simulink model "BetaMacs"  (R2023a)
settings: Solver=ode4  StartTime=0.0  StopTime=tsim  FixedStep=baseRate  RelTol=1e-6  AbsTol=1e-6
undefined symbols (not defined in the file): a1, a2, a3, b0, b1, b2, b3, baseRate, DiscIntNeverNeededParam, drop_states_ARM, drop_states_BLACK, drop_states_BLUE, drop_states_RED, F_Black_X_nominal, F_Black_Y_nominal, F_Blue_X_nominal, F_Blue_Y_nominal, F_red_X_nominal, F_red_Y_nominal, F_thrusters_BLACK, F_thrusters_BLUE, F_thrusters_RED, Gamma1_el, Gamma1_sh, Gamma1_wr, Gamma2_el, Gamma2_sh, Gamma2_wr, Gamma3_el, Gamma3_sh, Gamma3_wr, Gamma4_el, Gamma4_sh, Gamma4_wr, Gamma5_el, Gamma5_sh, Gamma5_wr, Gamma6_el, Gamma6_sh, Gamma6_wr, home_states_BLACK, home_states_BLUE, home_states_RED, IBLACK, IBLUE, IDIST, IEE, init_states_BLACK, init_states_BLUE, init_states_RED, IPROX, IRED, Kd_elarm, Kd_sharm, Kd_tb, Kd_tblue, Kd_tr, Kd_wrarm, Kd_xb, Kd_xblue ... (+48)
libraries: nvidiaSharedBlocks x9, MainLibrary x4, dspsigops x4, simulink x1
(part 11 of 11)

== matlab function BetaMacs/Thruster Control Code/Change RED Behavior/Calculate Thruster ON//OFF/MATLAB Function6 ==
  data: H output; thruster_dist2CG_RED parameter; F_red_X_nominal parameter; theta_1 input; theta_2 input; theta_3 input; mRED parameter; thrust_decay_factor input; F_red_Y_nominal parameter; mPROX parameter; mDIST parameter; mEE parameter; Phi parameter; b0 parameter; a1 parameter; b1 parameter; a2 parameter; b2 parameter; a3 parameter; b3 parameter
function H   = MakeHWithArmAndDecay(thruster_dist2CG_RED,F_red_X_nominal, theta_1, theta_2, theta_3,  mRED, thrust_decay_factor, F_red_Y_nominal, mPROX, mDIST, mEE, Phi, b0, a1, b1, a2, b2, a3, b3)
    
    link1_com_x = b0*cos(Phi) + a1*cos(pi/2 + theta_1);
    link1_com_y = b0*sin(Phi) + a1*sin(pi/2 + theta_1);
    
    link2_com_x = link1_com_x + b1*cos(pi/2 + theta_1) + a2*cos(pi/2 + theta_1 + theta_2);
    link2_com_y = link1_com_y + b1*sin(pi/2 + theta_1) + a2*sin(pi/2 + theta_1 + theta_2);
    
    link3_com_x = link2_com_x + b2*cos(pi/2 + theta_1 + theta_2) + a3*cos(pi/2 + theta_1 + theta_2 + theta_3);
    link3_com_y = link2_com_y + b2*sin(pi/2 + theta_1 + theta_2) + a3*sin(pi/2 + theta_1 + theta_2 + theta_3);
    
    delta_com_due_to_arm_x = (mPROX*link1_com_x + mDIST*link2_com_x + mEE*link3_com_x)/(mRED + mPROX + mDIST + mEE)*1000; % [mm]
    delta_com_due_to_arm_y = (mPROX*link1_com_y + mDIST*link2_com_y + mEE*link3_com_y)/(mRED + mPROX + mDIST + mEE)*1000; % [mm]
    
    adjusted_thruster_dist2CG_RED = [thruster_dist2CG_RED(1)-delta_com_due_to_arm_y;
                                     thruster_dist2CG_RED(2)-delta_com_due_to_arm_y;
                                     thruster_dist2CG_RED(3)-delta_com_due_to_arm_x;
                                     thruster_dist2CG_RED(4)-delta_com_due_to_arm_x;
                                     thruster_dist2CG_RED(5)+delta_com_due_to_arm_y;
                                     thruster_dist2CG_RED(6)+delta_com_due_to_arm_y;
                                     thruster_dist2CG_RED(7)+delta_com_due_to_arm_x;
                                     thruster_dist2CG_RED(8)+delta_com_due_to_arm_x];
                                 
    
    
    Vec1 = [ -1
             -1
              0 
              0
              1
              1
              0
              0 ];
          
    Vec2 = [  0
              0
              1
              1
              0
              0
             -1
             -1 ];
         
    Vec3 = adjusted_thruster_dist2CG_RED./1000;
    
    Mat1 = [Vec1, Vec2, Vec3]';
    
    F_thrusters_RED = [F_red_X_nominal*thrust_decay_factor; F_red_X_nominal*thrust_decay_factor; F_red_Y_nominal*thrust_decay_factor; F_red_Y_nominal*thrust_decay_factor; F_red_X_nominal*thrust_decay_factor; F_red_X_nominal*thrust_decay_factor; F_red_Y_nominal*thrust_decay_factor; F_red_Y_nominal*thrust_decay_factor];
    
    Mat2 = diag((F_thrusters_RED./2));
    
    H    = Mat1*Mat2;

end

== matlab function BetaMacs/Phase #3: Experiment/Change BLACK Behavior/Sub-Phase #2 /Hough Control/MATLAB Function3 ==
  data: z input; Ox output
function Ox    = C3( z )
%C3 gives the rotation matrix about the z-axis for an angle 'z'
%   z - the angle about the z-axis which you rotate
%   A - the rotation matrix

Ox = [cos(z) sin(z); -sin(z) cos(z)]*[1;0];
end

== matlab function BetaMacs/Phase #3: Experiment/Change BLACK Behavior/Sub-Phase #2 /Hough Control/MATLAB Function4 ==
  data: Oy input; e_out output; e_in input
function e_out = fcn(Oy, e_in)

a = sign(Oy'*e_in);
e_out = -a*norm(e_in);

== matlab function BetaMacs/Phase #3: Experiment/Change BLACK Behavior/Sub-Phase #3 /Hough Control/MATLAB Function4 ==
  data: Oy input; e_out output; e_in input
function e_out = fcn(Oy, e_in)

a = sign(Oy'*e_in);
e_out = -a*norm(e_in);

== matlab function BetaMacs/Phase #3: Experiment/Change RED Behavior/Sub-Phase #2 /MATLAB Function ==
  data: t input; x output; xLength parameter
function x = fcn(t, xLength)

x = 0.9*cos((0.03490659)*t) + xLength/2;

end

== matlab function BetaMacs/Phase #3: Experiment/Change BLUE Behavior/Sub-Phase #4/BLUE_Rz Desired/Wrap/MATLAB Function ==
  data: u input; wrappedAngle output
function wrappedAngle = wrapAngle(u)

wrappedAngle = atan2(sin(u),cos(u));

end

== matlab function BetaMacs/Phase #3: Experiment/Change RED Behavior/Sub-Phase #2 /MATLAB Function1 ==
  data: t input; y output; yLength parameter
function y = fcn(t, yLength)

y = 0.85*sin((0.03490659)*t) + yLength/2;

end

== matlab function BetaMacs/Phase #3: Experiment/Change RED Behavior/Sub-Phase #3 /Hough Control/MATLAB Function2 ==
  data: Oy output; z input; Ox output
function [Oy, Ox]   = C3( z )
%C3 gives the rotation matrix about the z-axis for an angle 'z'
%   z - the angle about the z-axis which you rotate
%   A - the rotation matrix

Ox = [cos(z) sin(z); -sin(z) cos(z)]*[1;0];
Oy = [cos(z) sin(z); -sin(z) cos(z)]*[0;1];
end

== matlab function BetaMacs/Phase #3: Experiment/Change RED Behavior/Sub-Phase #3 /Hough Control/MATLAB Function3 ==
  data: z input; Ox output
function Ox    = C3( z )
%C3 gives the rotation matrix about the z-axis for an angle 'z'
%   z - the angle about the z-axis which you rotate
%   A - the rotation matrix

Ox = [cos(z) sin(z); -sin(z) cos(z)]*[1;0];
end

== matlab function BetaMacs/Phase #3: Experiment/Change RED Behavior/Sub-Phase #3 /Hough Control/MATLAB Function4 ==
  data: Oy input; e_out output; e_in input
function e_out = fcn(Oy, e_in)

a = sign(Oy'*e_in);
e_out = -a*norm(e_in);

== matlab function BetaMacs/Phase #3: Experiment/Change RED Behavior/Sub-Phase #3 /MATLAB Function ==
  data: t input; x output; xLength parameter
function x = fcn(t, xLength)

x = 0.9*cos((0.03490659)*t) + xLength/2;

end

== matlab function BetaMacs/Phase #3: Experiment/Change RED Behavior/Sub-Phase #3 /MATLAB Function1 ==
  data: t input; y output; yLength parameter
function y = fcn(t, yLength)

y = 0.85*sin((0.03490659)*t) + yLength/2;

end

== matlab function BetaMacs/Phase #3: Experiment/Change BLACK Behavior/Sub-Phase #3 /BLACK_Rz Desired/Wrap1/MATLAB Function ==
  data: u input; wrappedAngle output
function wrappedAngle = wrapAngle(u)

wrappedAngle = atan2(sin(u),cos(u));

end

== matlab function BetaMacs/Phase #3: Experiment/Change BLACK Behavior/Sub-Phase #3 /Hough Control/MATLAB Function2 ==
  data: Oy output; z input; Ox output
function [Oy, Ox]   = C3( z )
%C3 gives the rotation matrix about the z-axis for an angle 'z'
%   z - the angle about the z-axis which you rotate
%   A - the rotation matrix

Ox = [cos(z) sin(z); -sin(z) cos(z)]*[1;0];
Oy = [cos(z) sin(z); -sin(z) cos(z)]*[0;1];
end

== matlab function BetaMacs/Phase #3: Experiment/Change BLACK Behavior/Sub-Phase #3 /Hough Control/MATLAB Function3 ==
  data: z input; Ox output
function Ox    = C3( z )
%C3 gives the rotation matrix about the z-axis for an angle 'z'
%   z - the angle about the z-axis which you rotate
%   A - the rotation matrix

Ox = [cos(z) sin(z); -sin(z) cos(z)]*[1;0];
end

== matlab function BetaMacs/Phase #5: Hold Home/Change BLACK Behavior/Hough Control/MATLAB Function2 ==
  data: Oy output; z input; Ox output
function [Oy, Ox]   = C3( z )
%C3 gives the rotation matrix about the z-axis for an angle 'z'
%   z - the angle about the z-axis which you rotate
%   A - the rotation matrix

Ox = [cos(z) sin(z); -sin(z) cos(z)]*[1;0];
Oy = [cos(z) sin(z); -sin(z) cos(z)]*[0;1];
end

== matlab function BetaMacs/Phase #3: Experiment/Change BLUE Behavior/Sub-Phase #1/MATLAB Function2 ==
  data: t input; x output; xLength parameter
function x = fcn(t, xLength)

x = -0.85*cos((0.03490659)*t) + xLength/2;

end

== matlab function BetaMacs/Phase #3: Experiment/Change BLACK Behavior/Sub-Phase #1/Hough Control/MATLAB Function4 ==
  data: Oy input; e_out output; e_in input
function e_out = fcn(Oy, e_in)

a = sign(Oy'*e_in);
e_out = -a*norm(e_in);

== matlab function BetaMacs/Phase #3: Experiment/Change BLUE Behavior/Sub-Phase #1/MATLAB Function3 ==
  data: t input; y output; yLength parameter
function y = fcn(t, yLength)

y = -0.85*sin((0.03490659)*t) + yLength/2;

end

== matlab function BetaMacs/PhaseSpace Camera Code/Use Hardware to Obtain States/MATLAB Function ==
  data: StartClock output; RedReceiving input; BlackReceiving input; BlueReceiving input; platformSelection parameter
function StartClock = CheckForSync(RedReceiving, BlackReceiving, BlueReceiving, platformSelection)
        
    StartClock = 0;
    
    if (platformSelection == 1)
        
        if RedReceiving == 1

            StartClock = 1;

        else

            StartClock = 0;

        end
        
    elseif (platformSelection == 2)
        
        if BlackReceiving == 1

            StartClock = 1;

        else

            StartClock = 0;

        end  
        
    elseif (platformSelection == 3)
        
        if RedReceiving == 1 && BlackReceiving == 1

            StartClock = 1;

        else

            StartClock = 0;

        end    
        
    elseif (platformSelection == 4)
        
        if RedReceiving == 1 && BlackReceiving == 1

            StartClock = 1;

        else

            StartClock = 0;

        end
        
    elseif (platformSelection == 5)
        
        if RedReceiving == 1

            StartClock = 1;

        else

            StartClock = 0;

        end
        
    elseif (platformSelection == 6)
        
        if BlueReceiving == 1

            StartClock = 1;

        else

            StartClock = 0;

        end
        
    elseif (platformSelection == 7)
        
        if RedReceiving == 1 && BlueReceiving == 1

            StartClock = 1;

        else

            StartClock = 0;

        end
        
    elseif (platformSelection == 8)
        
        if RedReceiving == 1 && BlackReceiving == 1 && BlueReceiving == 1

            StartClock = 1;

        else

            StartClock = 0;

        end
        
    elseif (platformSelection == 9)
        
        if BlackReceiving == 1 && BlueReceiving == 1

            StartClock = 1;

        else

            StartClock = 0;

        end
                           
    elseif (platformSelection == 10)
        
        if RedReceiving == 1 && BlueReceiving == 1

            StartClock = 1;

        else

            StartClock = 0;

        end
        
    elseif (platformSelection == 11)
        
        if RedReceiving == 1 && BlackReceiving == 1 && BlueReceiving == 1

            StartClock = 1;

        else

            StartClock = 0;

        end
        
    end



end
